simulink model "mainEthan"  (R2023b)
settings: Solver=ode113  StartTime=tstart  StopTime=tend  RelTol=relTol  AbsTol=absTol
values from neighbouring files (symbols this model uses):
  DCM_initial = targetDCM([26321453.5527815,	-132781955.130633,	-57571626.5531097]', R_princ)    [EulerEquations.m]    (also in main_script.m)
  inertia_p = [85.075, 0, 0; 0, 85.075, 0; 0, 0, 120.2515]    [omega_dot.m]
  omega_init = [0; 0; 0.01]    [EulerEquations.m]    (also in main_script.m)
  state_ECI_init = [R_PQW_IJK*state_PQW_init(1:3)';R_PQW_IJK*state_PQW_init(4:6)']    [OrbitPropagation.m]
  theta = UT1_to_theta(UT1)    [EulerEquations.m]    (also in UT1_to_theta.m = rotz(-GMST*180/pi); main_script.m)
  tstart = 0    [EulerEquations.m]    (also in main_script.m)
  UT1 = [1,25,2004,00]    [EulerEquations.m]    (also in main_script.m)
undefined symbols (not defined in the file or in its folder): A, A_star, I_w, max_dipole, max_wheel_om, max_wheel_torque, omega_w_init, R_princ
libraries: simulink x4, dspmathops x3, aerolibatmos2 x1, matrix_library x1
(part 1 of 2)
settings Model: Creator=Anna  LastModifiedBy=Anna

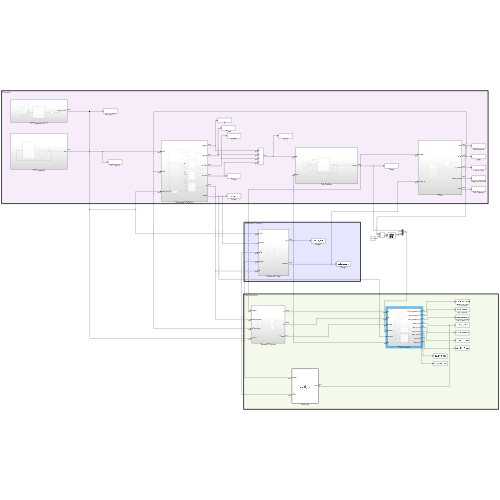
[thumbnail: Simulink's stored preview of the top-level diagram]
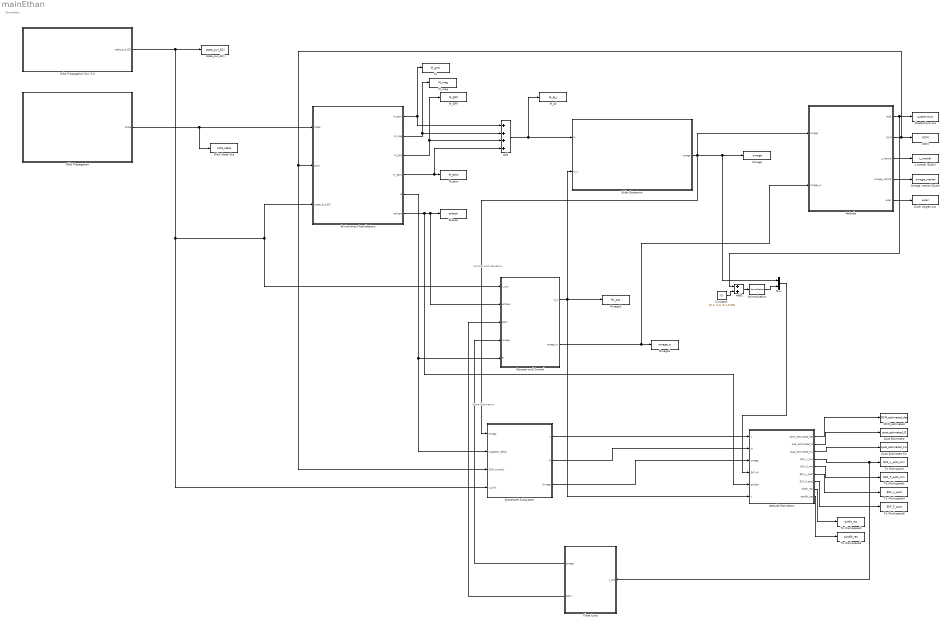
== system mainEthan ==
  note: Control and Actuation
  note: Simulation
  note: State Estimation
  Actuator and Control : Subsystem
  Add : Sum  Inputs=++++
  Add1 : Sum
  Attitude : Subsystem
  Attitude Estimation : Subsystem
  Close Loop : MATLAB Function  TreatAsAtomicUnit=on
  Constant : Constant  Value=[0.1, 0.2, 0.1,0.05]
  DCM : ToWorkspace  VariableName=DCM  SaveFormat=Timeseries  SampleTime=-1
  DCM_estimated : ToWorkspace  VariableName=DCM_estimated_det  SaveFormat=Timeseries  SampleTime=-1
      settings: Save2DSignal=2-D array (concatenate along first dimension)
  Eclipse : ToWorkspace  VariableName=eclipse  SaveFormat=Timeseries  SampleTime=-1
  Environment Petrubations : Subsystem
  Euler Angles out : ToWorkspace  VariableName=euler  SaveFormat=Timeseries  SampleTime=-1
  Euler Equations : Subsystem
  L inertial (Euler) : ToWorkspace  VariableName=L_inertial  SaveFormat=Timeseries  SampleTime=-1
  M : ToWorkspace  VariableName=M_grav  SaveFormat=Timeseries  SampleTime=-1
      settings: Save2DSignal=2-D array (concatenate along first dimension)
  M_All : ToWorkspace  VariableName=M_ALL  SaveFormat=Timeseries  SampleTime=-1
      settings: Save2DSignal=2-D array (concatenate along first dimension)
  M_SRP : ToWorkspace  VariableName=M_SRP  SaveFormat=Timeseries  SampleTime=-1
      settings: Save2DSignal=2-D array (concatenate along first dimension)
  M_aero : ToWorkspace  VariableName=M_aero  SaveFormat=Timeseries  SampleTime=-1
      settings: Save2DSignal=2-D array (concatenate along first dimension)
  M_mag : ToWorkspace  VariableName=M_mag  SaveFormat=Timeseries  SampleTime=-1
      settings: Save2DSignal=2-D array (concatenate along first dimension)
  Mux : Mux  Inputs=2
  Normalization : dspmathops/Normalization  NormType=Squared 2-norm  Bias=1e-10  NormOver=Each column  Dimension=1  roundingMode=Floor  overflowMode=off  accumDataTypeStr=Inherit: Same as product output  accumLastDataTypeStr=Inherit: Same as product output  outputDataTypeStr=Inherit: Same as product output  outputMin=[]  outputMax=[]  outputLastDataTypeStr=Inherit: Same as product output
  Omega : ToWorkspace  VariableName=omega  SaveFormat=Timeseries  SampleTime=-1
      settings: Save2DSignal=2-D array (concatenate along first dimension)
  Omega inertial (Euler) : ToWorkspace  VariableName=omega_inertial  SaveFormat=Timeseries  SampleTime=-1
  Omega1 : ToWorkspace  VariableName=omega_w  SaveFormat=Timeseries  SampleTime=-1
      settings: Save2DSignal=2-D array (concatenate along first dimension)
  Omega2 : ToWorkspace  VariableName=Mc_act  SaveFormat=Timeseries  SampleTime=-1
      settings: Save2DSignal=2-D array (concatenate along first dimension)
  Orbit Propagation : Subsystem
  Orbit Propagation Sun 3.0 : Subsystem
  Orbit State Out : ToWorkspace  VariableName=orbit_state  SaveFormat=Timeseries  SampleTime=-1
  Quat Estimated : ToWorkspace  VariableName=quat_estimated_Q  SaveFormat=Timeseries  SampleTime=-1
  Quat Estimated Kin : ToWorkspace  VariableName=quat_estimated_kin  SaveFormat=Timeseries  SampleTime=-1
  Quaternions out : ToWorkspace  VariableName=quaternions  SaveFormat=Timeseries  SampleTime=-1
  Spacecraft Subsystem : Subsystem
  To Workspace : ToWorkspace  VariableName=EKF_x_post_min  SaveFormat=Timeseries  SampleTime=-1
  To Workspace1 : ToWorkspace  VariableName=EKF_P_post_min  SaveFormat=Timeseries  SampleTime=-1
  To Workspace2 : ToWorkspace  VariableName=prefit_res  SaveFormat=Timeseries  SampleTime=-1
  To Workspace3 : ToWorkspace  VariableName=postfit_res  SaveFormat=Timeseries  SampleTime=-1
  To Workspace4 : ToWorkspace  VariableName=EKF_x_post  SaveFormat=Timeseries  SampleTime=-1
  To Workspace5 : ToWorkspace  VariableName=EKF_P_post  SaveFormat=Timeseries  SampleTime=-1
  state_sun_ECI : ToWorkspace  VariableName=state_sun_ECI  SaveFormat=Timeseries  SampleTime=-1
  wires:
  Environment Petrubations/2(M_mag) -> M_mag/1, Add/2
  Orbit Propagation/1(state) -> Orbit State Out/1, Environment Petrubations/1(state)
  Add/1 -> Euler Equations/1(M), M_All/1
  Environment Petrubations/3(M_SRP) -> M_SRP/1, Add/3
  Environment Petrubations/4(M_aero) -> Add/4, M_aero/1
  Orbit Propagation Sun 3.0/1(state_sun_ECI) -> Spacecraft Subsystem/4(r_sun1), Environment Petrubations/3(state_Sun_ECI), Actuator and Control/1(r_sun), state_sun_ECI/1
  Spacecraft Subsystem/1(V) -> Attitude Estimation/1(V)
  Spacecraft Subsystem/2(M) -> Attitude Estimation/2(M)
  Environment Petrubations/5(B) -> Spacecraft Subsystem/2(magnetic_field1), Actuator and Control/5(B)
  Attitude Estimation/1(DCM_estimated_det) -> DCM_estimated/1
  Attitude Estimation/2(quat_estimated_Q) -> Quat Estimated/1
  Attitude Estimation/3(quat_estimated_kin) -> Quat Estimated Kin/1
  Spacecraft Subsystem/3(Omega) -> Attitude Estimation/3(omega)
  Attitude Estimation/5(EKF_P_min) -> To Workspace1/1
  Attitude Estimation/4(EKF_x_min) -> To Workspace/1, Close Loop/1(x_est)
  Mux/1 -> Attitude Estimation/4(EKF x0)
  Attitude Estimation/7(EKF_P_post) -> To Workspace5/1
  Attitude Estimation/6(EKF_x_post) -> To Workspace4/1
  Environment Petrubations/6(eclipse) -> Attitude Estimation/5(" eclipse"), Actuator and Control/2(eclipse), Eclipse/1
  Attitude Estimation/8(prefit_res) -> To Workspace2/1
  Attitude Estimation/9(postfit_res) -> To Workspace3/1
  Normalization/1 -> Mux/2
  Add1/1 -> Normalization/1
  Constant/1 -> Add1/2
  Actuator and Control/1(M_c) -> Euler Equations/2(M_c), Omega2/1, Attitude Estimation/6(u)
  Actuator and Control/2(omega_w) -> Attitude/2(omega_w), Omega1/1
  Close Loop/1(omega) -> Actuator and Control/4(omega)
  Close Loop/2(DCM) -> Actuator and Control/3(DCM)
  Environment Petrubations/1(M_grav) -> Add/1, M/1
  Attitude/2(DCM) -> DCM/1, Spacecraft Subsystem/3(DCM current1), Environment Petrubations/2(DCM)
  Attitude/1(quat) -> Quaternions out/1, Add1/1
  Euler Equations/1(omega) -> Attitude/1(omega), Omega/1, Mux/1, Spacecraft Subsystem/1(omega)
  Attitude/3(L_inertial) -> L inertial (Euler)/1
  Attitude/4(omega_inertial) -> Omega inertial (Euler)/1
  Attitude/5(euler) -> Euler Angles out/1

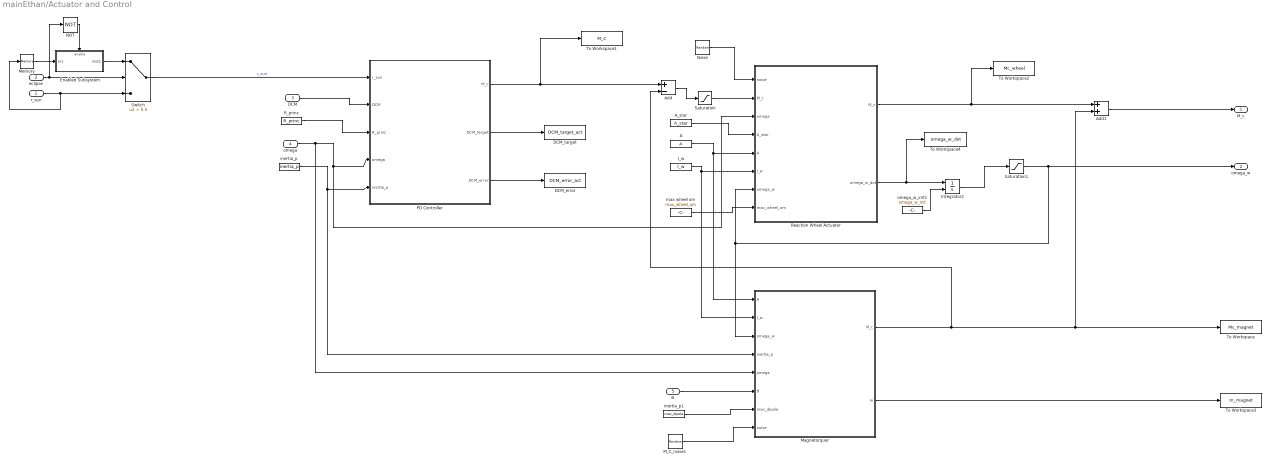
== system mainEthan/Actuator and Control ==
  r_sun : Inport
  eclipse : Inport  Port=2
  DCM : Inport  Port=3
  omega : Inport  Port=4
  B : Inport  Port=5
  A : Constant  Value=A
  A_star : Constant  Value=A_star
  Add : Sum  Inputs=+-
  Add1 : Sum
  DCM_error : ToWorkspace  VariableName=DCM_error_act  SaveFormat=Timeseries  SampleTime=-1
      settings: Save2DSignal=2-D array (concatenate along first dimension)
  DCM_target : ToWorkspace  VariableName=DCM_target_act  SaveFormat=Timeseries  SampleTime=-1
      settings: Save2DSignal=2-D array (concatenate along first dimension)
  Enabled Subsystem : Subsystem  TreatAsAtomicUnit=on
  I_w : Constant  Value=I_w
  Integrator2 : Integrator  InitialConditionSource=external  AbsoluteTolerance=absTol
  M_C_noise1 : RandomNumber  Variance=(0.00005/166)*2  Seed=[130,131,132]  SampleTime=0.1  VectorParams1D=off
  Magnetorquer : MATLAB Function  TreatAsAtomicUnit=on
  Memory : Memory  InitialCondition=[0;0;0]
  NOT : Logic  Operator=NOT  IconShape=distinctive  AllPortsSameDT=off  OutDataTypeStr=boolean
  Noise : RandomNumber  Variance=(0.00005/166)*2  Seed=[120,121,122, 123]  SampleTime=0.1  VectorParams1D=off
  PD Controller : MATLAB Function  TreatAsAtomicUnit=on
  R_princ : Constant  Value=R_princ
  Reaction Wheel Actuator : MATLAB Function  TreatAsAtomicUnit=on
  Saturation : Saturate  UpperLimit=max_wheel_torque  LowerLimit=-max_wheel_torque
  Saturation1 : Saturate  UpperLimit=max_wheel_om  LowerLimit=-max_wheel_om
  Switch : Switch  Criteria=u2 > Threshold  Threshold=0.5  SaturateOnIntegerOverflow=off  InputSameDT=off
  To Workspace : ToWorkspace  VariableName=Mc_magnet  SaveFormat=Timeseries  SampleTime=-1
  To Workspace1 : ToWorkspace  VariableName=M_C  SaveFormat=Timeseries  SampleTime=-1
  To Workspace2 : ToWorkspace  VariableName=Mc_wheel  SaveFormat=Timeseries  SampleTime=-1
  To Workspace3 : ToWorkspace  VariableName=m_magnet  SaveFormat=Timeseries  SampleTime=-1
  To Workspace4 : ToWorkspace  VariableName=omega_w_dot  SaveFormat=Timeseries  SampleTime=-1
  inertia_p : Constant  Value=inertia_p
  inertia_p1 : Constant  Value=max_dipole
  max wheel om : Constant  Value=max_wheel_om
  omega_w_init1 : Constant  Value=omega_w_init  VectorParams1D=off
  M_c : Outport
  omega_w : Outport  Port=2
  wires:
  omega_w_init1/1 -> Integrator2/2
  PD Controller/2(DCM_target) -> DCM_target/1
  omega/1 -> Reaction Wheel Actuator/3(omega), PD Controller/4(omega), Magnetorquer/5(omega)
  R_princ/1 -> PD Controller/3(R_princ)
  inertia_p/1 -> Magnetorquer/4(inertia_p), PD Controller/5(inertia_p)
  DCM/1 -> PD Controller/2(DCM)
  A_star/1 -> Reaction Wheel Actuator/4(A_star)
  PD Controller/3(DCM_error) -> DCM_error/1
  Reaction Wheel Actuator/2(omega_w_dot) -> To Workspace4/1, Integrator2/1
  Integrator2/1 -> Saturation1/1
  I_w/1 -> Reaction Wheel Actuator/6(I_w), Magnetorquer/2(I_w)
  A/1 -> Magnetorquer/1(A), Reaction Wheel Actuator/5(A)
  B/1 -> Magnetorquer/6(B)
  Magnetorquer/2(m) -> To Workspace3/1
  Switch/1 -> PD Controller/1(r_sun)  "r_sun"
  r_sun/1 -> Memory/1, Switch/3
  eclipse/1 -> NOT/1, Switch/2
  Memory/1 -> Enabled Subsystem/1(In1)
  Enabled Subsystem/1(Out1) -> Switch/1
  NOT/1 -> Enabled Subsystem/Enable
  PD Controller/1(M_c) -> Add/1, To Workspace1/1
  Saturation/1 -> Reaction Wheel Actuator/2("M_c ")
  Saturation1/1 -> omega_w/1, Magnetorquer/3(omega_w), Reaction Wheel Actuator/7(omega_w)
  max wheel om/1 -> Reaction Wheel Actuator/8(max_wheel_om)
  Add/1 -> Saturation/1
  Add1/1 -> M_c/1
  Reaction Wheel Actuator/1(M_c) -> To Workspace2/1, Add1/1
  Magnetorquer/1(M_c) -> Add/2, Add1/2, To Workspace/1
  inertia_p1/1 -> Magnetorquer/7(max_dipole)
  Noise/1 -> Reaction Wheel Actuator/1(noise)
  M_C_noise1/1 -> Magnetorquer/8(noise)

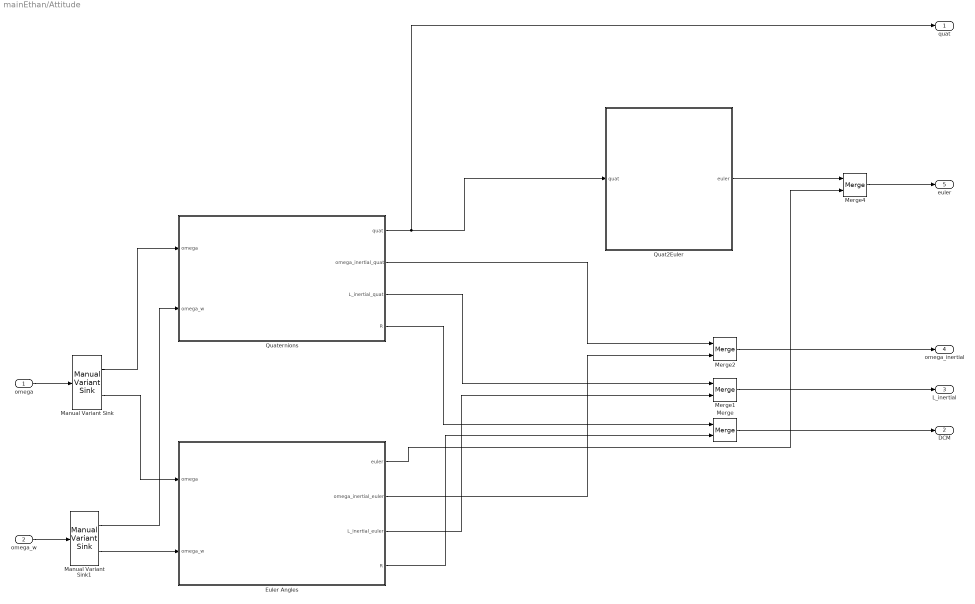
== system mainEthan/Attitude ==
  omega : Inport
  omega_w : Inport  Port=2
  Euler Angles : Subsystem
  Manual Variant Sink : simulink/Signal Routing/Manual Variant Sink  NumChoices=2  LabelModeActiveChoice=V_1
  Manual Variant Sink1 : simulink/Signal Routing/Manual Variant Sink  NumChoices=2  LabelModeActiveChoice=V_1
  Merge{,1..2,4} (4 alike) : Merge
  Quat2Euler : MATLAB Function  TreatAsAtomicUnit=on
  Quaternions : Subsystem
  quat : Outport
  DCM : Outport  Port=2
  L_inertial : Outport  Port=3
  omega_inertial : Outport  Port=4
  euler : Outport  Port=5
  wires:
  Merge/1 -> DCM/1
  omega/1 -> Manual Variant Sink/1
  omega_w/1 -> Manual Variant Sink1/1
  Quaternions/1(quat) -> quat/1, Quat2Euler/1(quat)
  Euler Angles/1(euler) -> Merge4/2
  Euler Angles/3(L_inertial_euler) -> Merge1/2
  Quat2Euler/1(euler) -> Merge4/1
  Manual Variant Sink1/1 -> Quaternions/2(omega_w)
  Manual Variant Sink1/2 -> Euler Angles/2(omega_w)
  Euler Angles/4(R) -> Merge/2
  Manual Variant Sink/1 -> Quaternions/1(omega)
  Quaternions/4(R) -> Merge/1
  Quaternions/3(L_inertial_quat) -> Merge1/1
  Manual Variant Sink/2 -> Euler Angles/1(omega)
  Merge1/1 -> L_inertial/1
  Merge2/1 -> omega_inertial/1
  Merge4/1 -> euler/1
  Quaternions/2(omega_inertial_quat) -> Merge2/1
  Euler Angles/2(omega_inertial_euler) -> Merge2/2

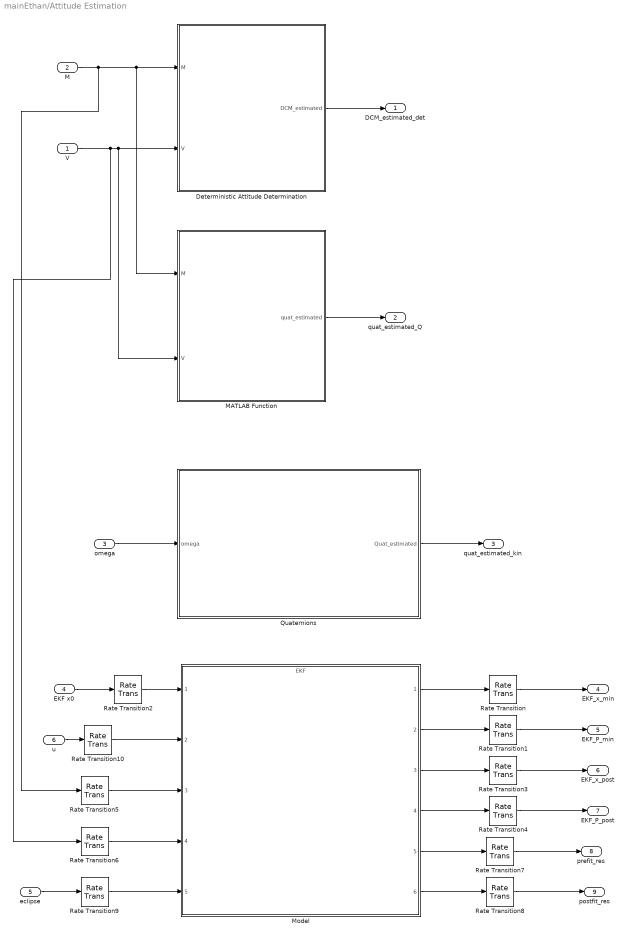
== system mainEthan/Attitude Estimation ==
  V : Inport
  M : Inport  Port=2
  omega : Inport  Port=3
  EKF x0 : Inport  Port=4
  " eclipse" : Inport  Port=5  PortDimensions=1
  u : Inport  Port=6
  Deterministic Attitude Determination : MATLAB Function  TreatAsAtomicUnit=on
  MATLAB Function : MATLAB Function  TreatAsAtomicUnit=on
  Model : ModelReference  ModelNameDialog=EKF.slx  SimulationMode=Normal  ModelReferenceVersion=1.144
  Quaternions : Subsystem
  Rate Transition{,1..10} (11 alike) : RateTransition
  DCM_estimated_det : Outport
  quat_estimated_Q : Outport  Port=2
  quat_estimated_kin : Outport  Port=3
  EKF_x_min : Outport  Port=4
  EKF_P_min : Outport  Port=5
  EKF_x_post : Outport  Port=6
  EKF_P_post : Outport  Port=7
  prefit_res : Outport  Port=8
  postfit_res : Outport  Port=9
  wires:
  Deterministic Attitude Determination/1(DCM_estimated) -> DCM_estimated_det/1
  MATLAB Function/1(quat_estimated) -> quat_estimated_Q/1
  M/1 -> Rate Transition5/1, MATLAB Function/1(M), Deterministic Attitude Determination/1(M)
  Quaternions/1(Quat_estimated) -> quat_estimated_kin/1
  V/1 -> Rate Transition6/1, MATLAB Function/2(V), Deterministic Attitude Determination/2(V)
  omega/1 -> Quaternions/1(omega)
  Model/1 -> Rate Transition/1
  Rate Transition/1 -> EKF_x_min/1
  Model/2 -> Rate Transition1/1
  Rate Transition1/1 -> EKF_P_min/1
  EKF x0/1 -> Rate Transition2/1
  Rate Transition2/1 -> Model/1
  Model/3 -> Rate Transition3/1
  Model/4 -> Rate Transition4/1
  Rate Transition4/1 -> EKF_P_post/1
  Rate Transition3/1 -> EKF_x_post/1
  Rate Transition5/1 -> Model/3
  Rate Transition6/1 -> Model/4
  Rate Transition7/1 -> prefit_res/1
  Model/5 -> Rate Transition7/1
  Rate Transition8/1 -> postfit_res/1
  Model/6 -> Rate Transition8/1
  Rate Transition9/1 -> Model/5
  " eclipse"/1 -> Rate Transition9/1
  Rate Transition10/1 -> Model/2
  u/1 -> Rate Transition10/1

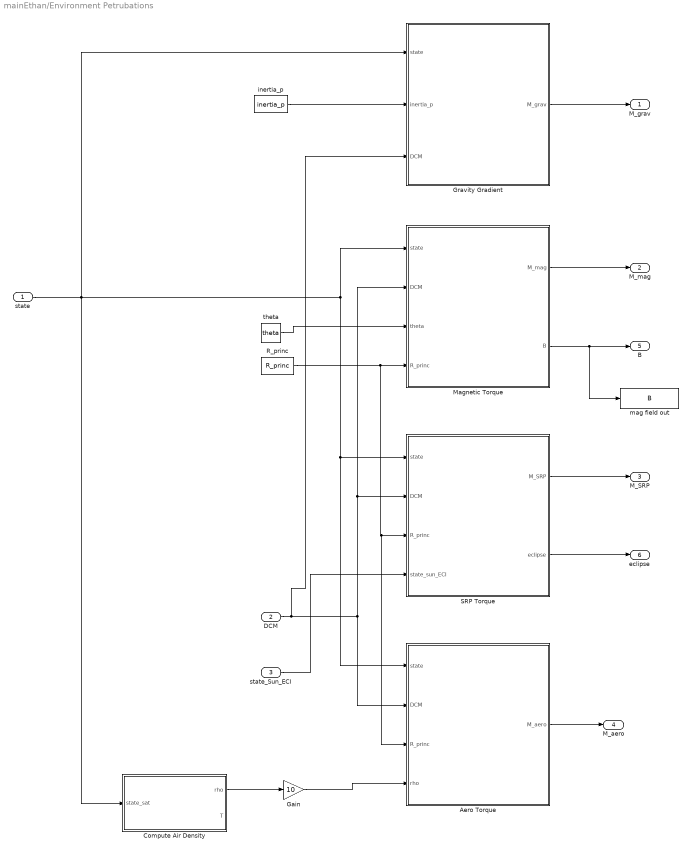
== system mainEthan/Environment Petrubations ==
  state : Inport
  DCM : Inport  Port=2
  state_Sun_ECI : Inport  Port=3
  Aero Torque : MATLAB Function  TreatAsAtomicUnit=on
  Compute Air Density : Subsystem
  Gain : Gain  Gain=10
  Gravity Gradient : MATLAB Function  TreatAsAtomicUnit=on
  Magnetic Torque : MATLAB Function  TreatAsAtomicUnit=on
  R_princ : Constant  Value=R_princ
  SRP Torque : MATLAB Function  TreatAsAtomicUnit=on
  inertia_p : Constant  Value=inertia_p
  mag field out : ToWorkspace  VariableName=B  SaveFormat=Timeseries  SampleTime=-1
  theta : Constant  Value=theta
  M_grav : Outport
  M_mag : Outport  Port=2
  M_SRP : Outport  Port=3
  M_aero : Outport  Port=4
  B : Outport  Port=5
  eclipse : Outport  Port=6
  wires:
  Magnetic Torque/1(M_mag) -> M_mag/1
  SRP Torque/1(M_SRP) -> M_SRP/1
  state/1 -> Magnetic Torque/1(state), Aero Torque/1(state), SRP Torque/1(state), Gravity Gradient/1(state), Compute Air Density/1(state_sat)
  DCM/1 -> Gravity Gradient/3(DCM), Aero Torque/2(DCM), Magnetic Torque/2(DCM), SRP Torque/2(DCM)
  theta/1 -> Magnetic Torque/3(theta)
  R_princ/1 -> Aero Torque/3(R_princ), SRP Torque/3(R_princ), Magnetic Torque/4(R_princ)
  state_Sun_ECI/1 -> SRP Torque/4(state_sun_ECI)
  Aero Torque/1(M_aero) -> M_aero/1
  SRP Torque/2(eclipse) -> eclipse/1
  Magnetic Torque/2(B) -> mag field out/1, B/1
  Gain/1 -> Aero Torque/4(rho)
  Compute Air Density/1(rho) -> Gain/1
  Gravity Gradient/1(M_grav) -> M_grav/1
  inertia_p/1 -> Gravity Gradient/2(inertia_p)

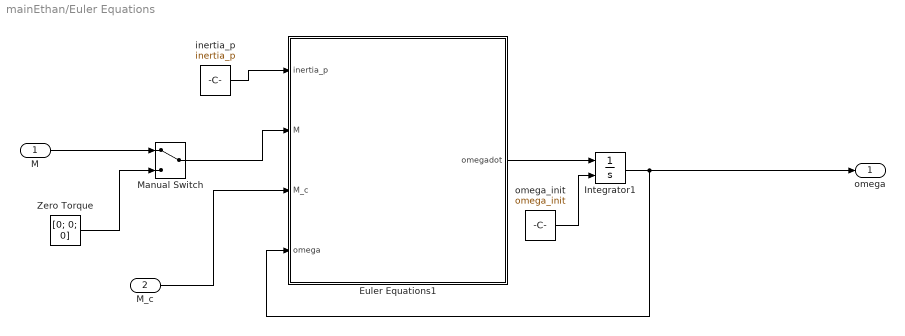
== system mainEthan/Euler Equations ==
  M : Inport
  M_c : Inport  Port=2
  Euler Equations1 : MATLAB Function  TreatAsAtomicUnit=on
  Integrator1 : Integrator  InitialConditionSource=external  AbsoluteTolerance=absTol
  Manual Switch : ManualSwitch
  Zero Torque : Constant  Value=[0; 0; 0]
  inertia_p : Constant  Value=inertia_p
  omega_init : Constant  Value=omega_init  VectorParams1D=off
  omega : Outport
  wires:
  inertia_p/1 -> Euler Equations1/1(inertia_p)
  Euler Equations1/1(omegadot) -> Integrator1/1
  Integrator1/1 -> omega/1, Euler Equations1/4(omega)
  omega_init/1 -> Integrator1/2
  Manual Switch/1 -> Euler Equations1/2(M)
  M/1 -> Manual Switch/1
  Zero Torque/1 -> Manual Switch/2
  M_c/1 -> Euler Equations1/3(M_c)

== system mainEthan/Orbit Propagation ==
  Integrator3 : Integrator  InitialConditionSource=external  AbsoluteTolerance=absTol
  Orbit Propagation1 : MATLAB Function  TreatAsAtomicUnit=on
  initial state ECI : Constant  Value=state_ECI_init
  state : Outport
  wires:
  initial state ECI/1 -> Integrator3/2
  Orbit Propagation1/1(statedot) -> Integrator3/1
  Integrator3/1 -> state/1, Orbit Propagation1/1(state)

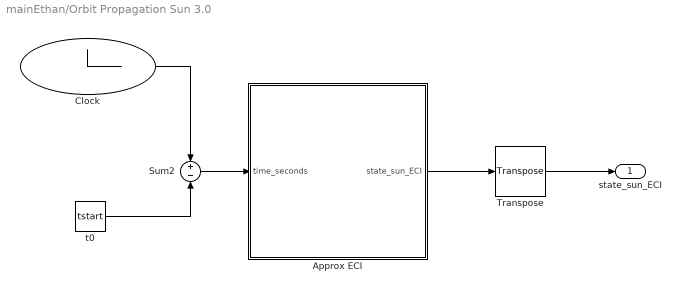
== system mainEthan/Orbit Propagation Sun 3.0 ==
  Approx ECI : MATLAB Function  TreatAsAtomicUnit=on
  Clock : Clock
  Sum2 : Sum  Inputs=+-
  Transpose : matrix_library/Transpose
  t0 : Constant  Value=tstart
  state_sun_ECI : Outport
  wires:
  Clock/1 -> Sum2/1
  t0/1 -> Sum2/2
  Sum2/1 -> Approx ECI/1(time_seconds)
  Transpose/1 -> state_sun_ECI/1
  Approx ECI/1(state_sun_ECI) -> Transpose/1

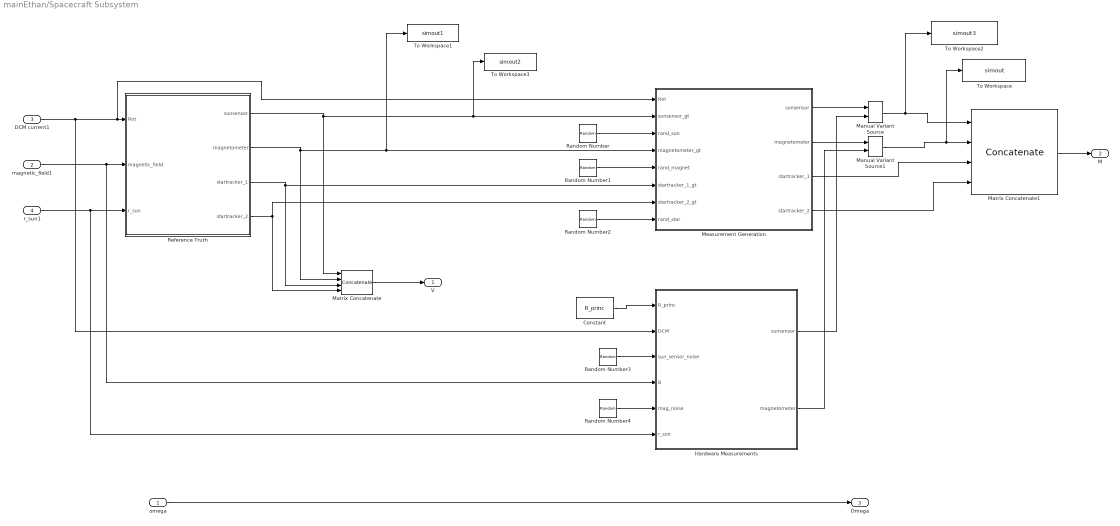
== system mainEthan/Spacecraft Subsystem ==
  omega : Inport
  magnetic_field1 : Inport  Port=2
  DCM current1 : Inport  Port=3
  r_sun1 : Inport  Port=4
  Constant : Constant  Value=R_princ
  Hardware Measurements : MATLAB Function  TreatAsAtomicUnit=on
  Manual Variant Source : simulink/Signal Routing/Manual Variant Source  NumChoices=2  LabelModeActiveChoice=V_2
  Manual Variant Source1 : simulink/Signal Routing/Manual Variant Source  NumChoices=2  LabelModeActiveChoice=V_2
  Matrix Concatenate : Concatenate  NumInputs=4  Mode=Multidimensional array  ConcatenateDimension=2
  Matrix Concatenate1 : Concatenate  NumInputs=4  Mode=Multidimensional array  ConcatenateDimension=2
  Measurement Generation : MATLAB Function  TreatAsAtomicUnit=on
  Random Number : RandomNumber  Variance=0.5  Seed=[80, 81]  SampleTime=0.1
  Random Number1 : RandomNumber  Variance=0.0075*65*10^-6  Seed=[70, 71, 72]  SampleTime=0.1
  Random Number2 : RandomNumber  Variance=5/3600  Seed=[0, 1,2,3,4,5,6,7,8,9,10,11,12,13,14; 15,16,17,18,19,20,21,22,23,24,25,26,27,28,29; 30, 31, 32,33,34,35,36,37,38,39,40,41,42,43,44;45,46,47,48,49,50,51,52,53,54,55,56,57,58,59]  SampleTime=0.1
  Random Number3 : RandomNumber  Variance=.0025  Seed=91  SampleTime=0.1
  Random Number4 : RandomNumber  Variance=100*((10^-6)/(10^-9))*12*10^-12  Seed=[95, 96, 97]  SampleTime=0.1
  Reference Truth : MATLAB Function  TreatAsAtomicUnit=on
  To Workspace : ToWorkspace  VariableName=simout  SaveFormat=Timeseries  SampleTime=-1
  To Workspace1 : ToWorkspace  VariableName=simout1  SaveFormat=Timeseries  SampleTime=-1
  To Workspace2 : ToWorkspace  VariableName=simout3  SaveFormat=Timeseries  SampleTime=-1
  To Workspace3 : ToWorkspace  VariableName=simout2  SaveFormat=Timeseries  SampleTime=-1
  V : Outport
  M : Outport  Port=2
  Omega : Outport  Port=3
  wires:
  r_sun1/1 -> Reference Truth/3(r_sun), Hardware Measurements/6(r_sun)
  magnetic_field1/1 -> Hardware Measurements/4(B), Reference Truth/2(magnetic_field)
  DCM current1/1 -> Hardware Measurements/2(DCM), Measurement Generation/1(Rot), Reference Truth/1(Rot)
  Matrix Concatenate1/1 -> M/1
  Matrix Concatenate/1 -> V/1
  Reference Truth/1(sunsensor) -> Matrix Concatenate/1, To Workspace3/1, Measurement Generation/2(sunsensor_gt)
  Reference Truth/3(startracker_1) -> Measurement Generation/6(startracker_1_gt), Matrix Concatenate/3
  Reference Truth/4(startracker_2) -> Measurement Generation/7(startracker_2_gt), Matrix Concatenate/4
  omega/1 -> Omega/1
  Random Number/1 -> Measurement Generation/3(rand_sun)
  Random Number1/1 -> Measurement Generation/5(rand_magnet)
  Random Number2/1 -> Measurement Generation/8(rand_star)
  Measurement Generation/4(startracker_2) -> Matrix Concatenate1/4
  Reference Truth/2(magnetometer) -> To Workspace1/1, Measurement Generation/4(magnetometer_gt), Matrix Concatenate/2
  Measurement Generation/3(startracker_1) -> Matrix Concatenate1/3
  Constant/1 -> Hardware Measurements/1(R_princ)
  Random Number3/1 -> Hardware Measurements/3(sun_sensor_noise)
  Manual Variant Source/1 -> To Workspace2/1, Matrix Concatenate1/1
  Measurement Generation/1(sunsensor) -> Manual Variant Source/1
  Hardware Measurements/1(sunsensor) -> Manual Variant Source/2
  Measurement Generation/2(magnetometer) -> Manual Variant Source1/1
  Manual Variant Source1/1 -> To Workspace/1, Matrix Concatenate1/2
  Hardware Measurements/2(magnetometer) -> Manual Variant Source1/2
  Random Number4/1 -> Hardware Measurements/5(mag_noise)

== system mainEthan/Actuator and Control/Enabled Subsystem ==
  In1 : Inport
  Enable : EnablePort
  Out1 : Outport
  wires:
  In1/1 -> Out1/1

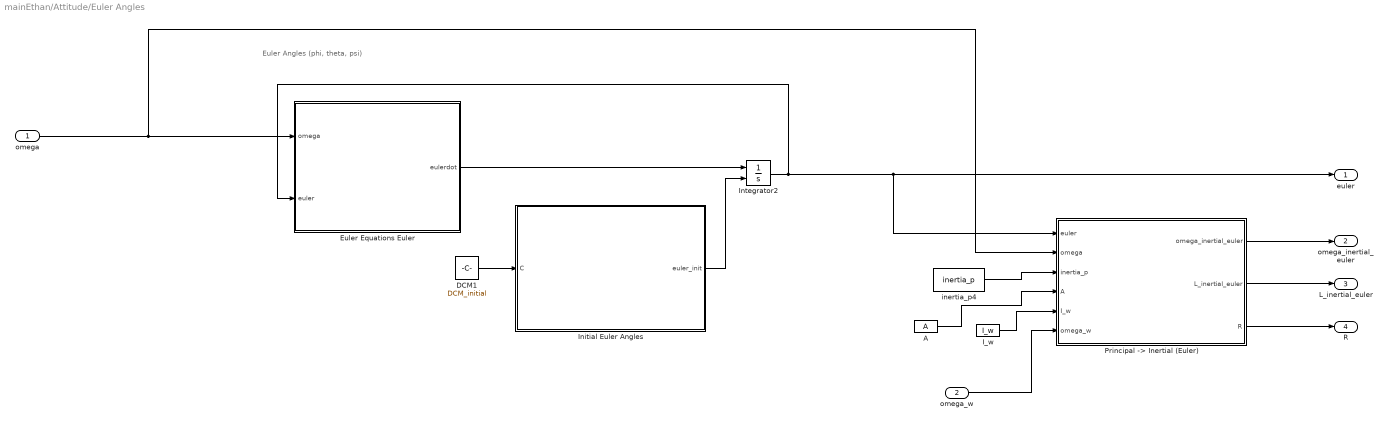
== system mainEthan/Attitude/Euler Angles ==
  note: Euler Angles (phi, theta, psi)
  omega : Inport
  omega_w : Inport  Port=2
  A : Constant  Value=A
  DCM1 : Constant  Value=DCM_initial
  Euler Equations Euler : MATLAB Function  TreatAsAtomicUnit=on
  I_w : Constant  Value=I_w
  Initial Euler Angles : MATLAB Function  TreatAsAtomicUnit=on
  Integrator2 : Integrator  InitialConditionSource=external  AbsoluteTolerance=absTol
  "Principal -> Inertial (Euler)" : MATLAB Function  TreatAsAtomicUnit=on
  inertia_p4 : Constant  Value=inertia_p
  euler : Outport
  omega_inertial_euler : Outport  Port=2
  L_inertial_euler : Outport  Port=3
  R : Outport  Port=4
  wires:
  "Principal -> Inertial (Euler)"/2(L_inertial_euler) -> L_inertial_euler/1
  Initial Euler Angles/1(euler_init) -> Integrator2/2
  "Principal -> Inertial (Euler)"/1(omega_inertial_euler) -> omega_inertial_euler/1
  "Principal -> Inertial (Euler)"/3(R) -> R/1
  Integrator2/1 -> euler/1, "Principal -> Inertial (Euler)"/1(euler), Euler Equations Euler/2(euler)
  Euler Equations Euler/1(eulerdot) -> Integrator2/1
  omega/1 -> "Principal -> Inertial (Euler)"/2(omega), Euler Equations Euler/1(omega)
  inertia_p4/1 -> "Principal -> Inertial (Euler)"/3(inertia_p)
  DCM1/1 -> Initial Euler Angles/1(C)
  omega_w/1 -> "Principal -> Inertial (Euler)"/6(omega_w)
  A/1 -> "Principal -> Inertial (Euler)"/4(A)
  I_w/1 -> "Principal -> Inertial (Euler)"/5(I_w)

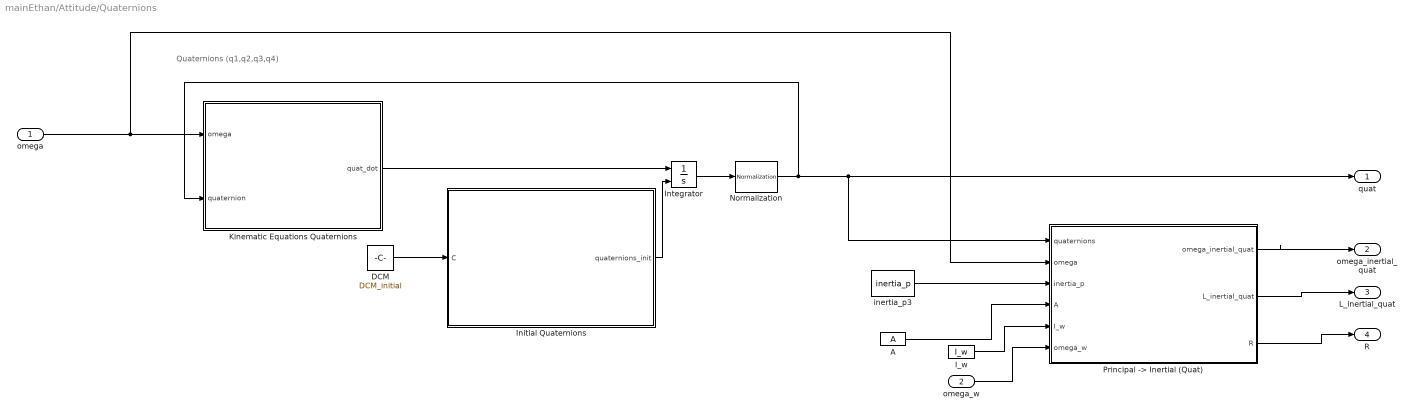
== system mainEthan/Attitude/Quaternions ==
  note: Quaternions (q1,q2,q3,q4)
  omega : Inport
  omega_w : Inport  Port=2
  A : Constant  Value=A
  DCM : Constant  Value=DCM_initial
  I_w : Constant  Value=I_w
  Initial Quaternions : MATLAB Function  TreatAsAtomicUnit=on
  Integrator : Integrator  InitialConditionSource=external  AbsoluteTolerance=absTol
  "Kinematic Equations Quaternions " : MATLAB Function  TreatAsAtomicUnit=on
  Normalization : dspmathops/Normalization  NormType=Squared 2-norm  Bias=1e-10  NormOver=Each column  Dimension=1  roundingMode=Floor  overflowMode=off  accumDataTypeStr=Inherit: Same as product output  accumLastDataTypeStr=Inherit: Same as product output  outputDataTypeStr=Inherit: Same as product output  outputMin=[]  outputMax=[]  outputLastDataTypeStr=Inherit: Same as product output
  "Principal -> Inertial (Quat)" : MATLAB Function  TreatAsAtomicUnit=on
  inertia_p3 : Constant  Value=inertia_p
  quat : Outport
  omega_inertial_quat : Outport  Port=2
  L_inertial_quat : Outport  Port=3
  R : Outport  Port=4
  wires:
  omega/1 -> "Kinematic Equations Quaternions "/1(omega), "Principal -> Inertial (Quat)"/2(omega)
  DCM/1 -> Initial Quaternions/1(C)
  "Principal -> Inertial (Quat)"/2(L_inertial_quat) -> L_inertial_quat/1
  "Kinematic Equations Quaternions "/1(quat_dot) -> Integrator/1
  "Principal -> Inertial (Quat)"/3(R) -> R/1
  Initial Quaternions/1(quaternions_init) -> Integrator/2
  Integrator/1 -> Normalization/1
  inertia_p3/1 -> "Principal -> Inertial (Quat)"/3(inertia_p)
  "Principal -> Inertial (Quat)"/1(omega_inertial_quat) -> omega_inertial_quat/1
  Normalization/1 -> quat/1, "Principal -> Inertial (Quat)"/1(quaternions), "Kinematic Equations Quaternions "/2(quaternion)
  A/1 -> "Principal -> Inertial (Quat)"/4(A)
  omega_w/1 -> "Principal -> Inertial (Quat)"/6(omega_w)
  I_w/1 -> "Principal -> Inertial (Quat)"/5(I_w)

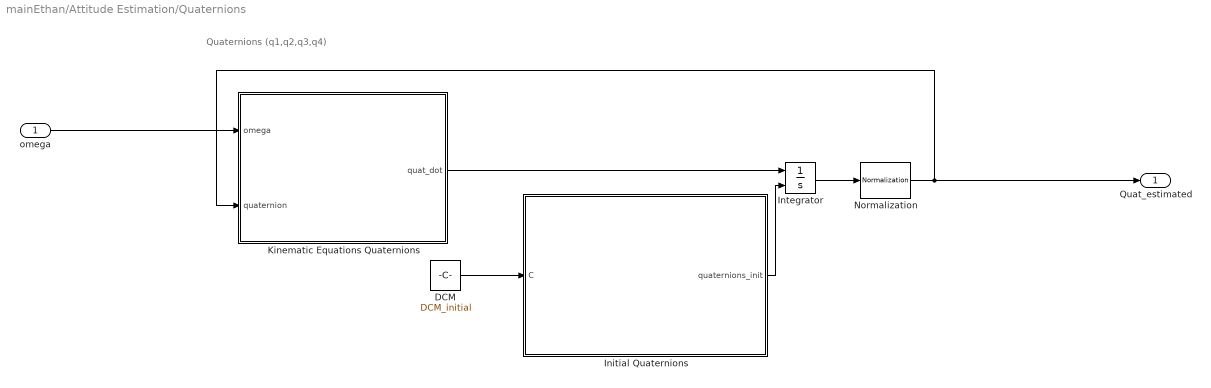
== system mainEthan/Attitude Estimation/Quaternions ==
  note: Quaternions (q1,q2,q3,q4)
  omega : Inport
  DCM : Constant  Value=DCM_initial
  Initial Quaternions : MATLAB Function  TreatAsAtomicUnit=on
  Integrator : Integrator  InitialConditionSource=external  AbsoluteTolerance=absTol
  "Kinematic Equations Quaternions " : MATLAB Function  TreatAsAtomicUnit=on
  Normalization : dspmathops/Normalization  NormType=Squared 2-norm  Bias=1e-10  NormOver=Each column  Dimension=1  roundingMode=Floor  overflowMode=off  accumDataTypeStr=Inherit: Same as product output  accumLastDataTypeStr=Inherit: Same as product output  outputDataTypeStr=Inherit: Same as product output  outputMin=[]  outputMax=[]  outputLastDataTypeStr=Inherit: Same as product output
  Quat_estimated : Outport
  wires:
  omega/1 -> "Kinematic Equations Quaternions "/1(omega)
  DCM/1 -> Initial Quaternions/1(C)
  "Kinematic Equations Quaternions "/1(quat_dot) -> Integrator/1
  Initial Quaternions/1(quaternions_init) -> Integrator/2
  Integrator/1 -> Normalization/1
  Normalization/1 -> Quat_estimated/1, "Kinematic Equations Quaternions "/2(quaternion)

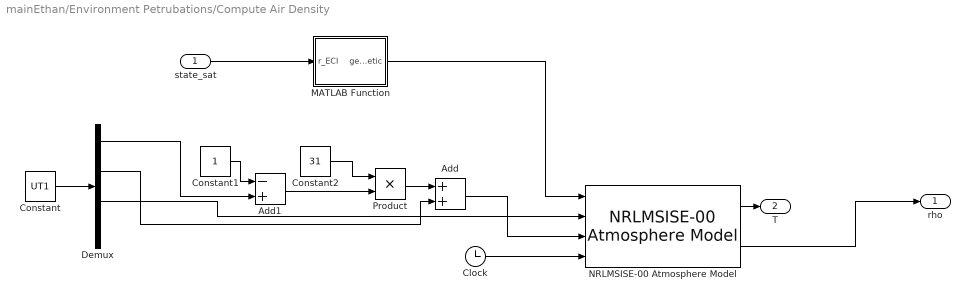
== system mainEthan/Environment Petrubations/Compute Air Density ==
  state_sat : Inport
  Add : Sum
  Add1 : Sum  Inputs=-+
  Clock : Clock
  Constant : Constant  Value=UT1
  Constant1 : Constant
  Constant2 : Constant  Value=31
  Demux : Demux
  MATLAB Function : MATLAB Function  TreatAsAtomicUnit=on
  NRLMSISE-00 Atmosphere Model : aerolibatmos2/NRLMSISE-00 Atmosphere Model  units=Metric (MKS)  lst_input=off  flux_ap_input=off  flags_input=Internal  flags=ones(1,23)  oxygen_in=off  action=Warning
  Product : Product
  rho : Outport
  T : Outport  Port=2
  wires:
  NRLMSISE-00 Atmosphere Model/1 -> T/1
  Demux/2 -> Add/2
  NRLMSISE-00 Atmosphere Model/2 -> rho/1
  Product/1 -> Add/1
  Add/1 -> NRLMSISE-00 Atmosphere Model/3
  MATLAB Function/1(geodetic) -> NRLMSISE-00 Atmosphere Model/1
  Demux/1 -> Add1/2
  Demux/3 -> NRLMSISE-00 Atmosphere Model/2
  Clock/1 -> NRLMSISE-00 Atmosphere Model/4
  Add1/1 -> Product/2
  Constant/1 -> Demux/1
  Constant2/1 -> Product/1
  state_sat/1 -> MATLAB Function/1(r_ECI)
  Constant1/1 -> Add1/1

== matlab function mainEthan/Orbit Propagation/Orbit Propagation1 ==
  data: statedot output; state input
%% return equations of motion
function statedot  = state_dot(state)
    mu = 398600.435436; %Earth centered orbit
    statedot = zeros(6, 1);
    statedot(1:3) = state(4:6);
    statedot(4:6) = -mu * state(1:3)/(norm(state(1:3))^3);
end

== matlab function mainEthan/Environment Petrubations/Gravity Gradient ==
  data: state input; inertia_p input; DCM input; M_grav output
%% return omega_dot (zero torque)
function M_grav  = gravity_gradient(state, inertia_p, DCM)
    mu = 398600.435436; %Earth centered orbit

    R_p = DCM * state(1:3);
    cx = R_p(1)/norm(R_p);
    cy = R_p(2)/norm(R_p);
    cz = R_p(3)/norm(R_p);

    M_grav = 3*mu/(norm(R_p)^3) *[(inertia_p(3,3) - inertia_p(2,2)) * cy * cz;
                    (inertia_p(1,1) - inertia_p(3,3)) * cz * cx;
                    (inertia_p(2,2) - inertia_p(1,1)) * cx * cy];
 
 
    %disp(norm(M))
end

== matlab function mainEthan/Attitude/Quat2Euler ==
  data: quat input; euler output

%% return euler angles from quaternions
function euler= quat2eul(quat)
    q0 = quat(4);
    q1 = quat(1);
    q2 = quat(2);
    q3 = quat(3);

    %123 singular for theta = 90 deg
    %phi = atan2(2*q2*q3 + 2*q0*q1, q3^2 - q2^2 - q1^2 + q0^2);
    %theta = -asin(2*q1*q3 - 2*q0*q2);
    %psi = atan2(2*q1*q2 + 2*q0*q3, q1^2 + q0^2 - q3^2 - q2^2);

    % %213 use when you rotate around y, singular for theta = 90
    phi = atan2(-2*q1*q3 + 2*q0*q2, q3^2 - q2^2 - q1^2 + q0^2);
    theta = asin(2*q2*q3 + 2*q0*q1);
    psi = atan2(-2*q1*q2 + 2*q0*q3, q2^2 - q3^2 + q0^2 - q1^2);

    %313 singular for theta = 0
    %phi = atan2(2*q1*q3 - 2*q0*q2, 2*q2*q3 + 2*q0*q1);
    %theta = acos(q3^2 - q2^2 - q1^2 + q0^2);
    %psi =atan2(2*q1*q3 + 2*q0*q2, -2*q2*q3 + 2*q0*q1);
    
    euler = [phi; theta; psi];

end

== matlab function mainEthan/Actuator and Control/PD Controller ==
  data: r_sun input; DCM input; R_princ input; M_c output; omega input; inertia_p input; DCM_target output; DCM_error output
%% return omega_dot (zero torque)
function [M_c, DCM_target, DCM_error]  = controller(r_sun, DCM, R_princ, omega, inertia_p)

    r_sun_norm = r_sun/norm(r_sun);

    %define that body x-axis will be in plane with body z-axis and r_sun
    %(perpendicular on r_sun)
    r_sun_projected = [r_sun_norm(1:2); 0];
    target_y_body = cross(r_sun_projected, r_sun_norm)./norm(cross(r_sun_projected, r_sun_norm));
    target_x_body = cross(target_y_body, r_sun_norm); %in plane

    %disp(dot(r_sun_norm, target_x_body)) %check that they are perependicular
    
    %construct target DCM in principal frame
    target_DCM = eye(3); %target DCM in principal frame
    target_DCM(1:3, 1) =  R_princ * target_x_body; %target attitude x-component principal frame
    target_DCM(1:3, 2) =  R_princ * target_y_body; %target attitude y-component principal frame
    target_DCM(1:3, 3) =  R_princ * r_sun_norm; %target attitude z-component principal frame

    DCM_target = target_DCM;
    DCM_error = DCM*DCM_target';
    n = 0.0011;
    kpx = 100*inertia_p(1,1)*n^2;
    kpy = 100*inertia_p(2,2)*n^2;
    kpz = 100*inertia_p(3,3)*n^2;

   

    kdx = 2 * 0.7 * inertia_p(1,1) * 100*n;
    kdy = 2 * 0.7 * inertia_p(2,2) * 100*n;
    kdz = 2 * 0.7 * inertia_p(3,3) * 100*n;

    
    % %Small Angle Approx
    % M_c = [0;0;0];
    % M_c(1) = - 0.5*kpx*(DCM_error(2,3) - DCM_error(3,2)) - kdx*omega(1);
    % M_c(2) = - 0.5*kpy*(DCM_error(1,3) - DCM_error(3,1)) - kdy*omega(2);
    % M_c(3) = - 0.5*kpz*(DCM_error(1,2) - DCM_error(2,1)) - kdz*omega(3);
    % 
    %213 seq
    alphay = atan2(-DCM_error(1, 3), DCM_error(3, 3));
    alphax = asin(DCM_error(2, 3));
    alphaz = atan2(-DCM_error(2, 1), DCM_error(2, 2));
    M_c = [0;0;0];
    M_c(1) = - kpx*alphax - kdx*omega(1);
    M_c(2) = - kpy*alphay- kdy*omega(2);
    M_c(3) = - kpz*alphaz - kdz*omega(3);

end

== matlab function mainEthan/Actuator and Control/Reaction Wheel Actuator ==
  data: noise input; M_c input; omega input; A_star input; A input; I_w input; omega_w input; M_c output; omega_w_dot output; max_wheel_om input
function [M_c, omega_w_dot] = RW_actuator(noise, M_c, omega, A_star, A, I_w, omega_w, max_wheel_om)
    L_w = I_w.*omega_w;
    L_w_dot = A_star * (- M_c - cross(omega,A*L_w)) + noise';
    omega_w_dot = L_w_dot./I_w;

    indices_pos_sat = (omega_w >= max_wheel_om) & (omega_w_dot > 0);
    indices_neg_sat = (omega_w <= -max_wheel_om) & (omega_w_dot < 0);
  
    omega_w_dot(indices_pos_sat | indices_neg_sat) = 0;
   

    M_c = - I_w  .* pinv(A_star) * omega_w_dot - cross(omega, A*L_w);
end

== matlab function mainEthan/Environment Petrubations/SRP Torque ==
  data: state input; DCM input; R_princ input; M_SRP output; state_sun_ECI input; eclipse output
function [M_SRP, eclipse] = SRP_torque(state, DCM, R_princ, state_sun_ECI)
    P = 1358/(3e8); % Solar Constant

    R = state(1:3)*1000; % State ECI
    R_unit = R./norm(R); % Unit State ECI
    R_E = 6378*1000; % Earth Radius

    R_Sun = state_sun_ECI; % Sun State ECI 
    R_Sun_unit = R_Sun./norm(R_Sun); % Unit Sun State ECI
    R_p_Sun = DCM * R_Sun; % Sun State Princ
    R_p_Sun_unit = R_p_Sun./norm(R_p_Sun); % Unit Sun State Princ

    M_SRP = [0;0;0];

    surface = struct('bary',[0,0,0],'size',0,'unit',[0,0,0]);

    % Eclipses
    psi = acos(dot(R_unit, R_Sun_unit));
    a_check = norm(R)*sin(psi);

    for surfacenum = 1:20
        if surfacenum == 1
            surface.bary = [-0.0129, -0.0019, 1.0022]; % Converted from cm to m
            surface.size = 0.866025; % Converted from cm² to m²
            surface.unit = [0, 0, 1];
        end
        if surfacenum == 2
            surface.bary = [-0.0129, -0.0019, -0.6008]; % Converted from cm to m
            surface.size = 0.866025; % Converted from cm² to m²
            surface.unit = [0, 0, -1];
        end
        if surfacenum == 3
            surface.bary = [0.4871, -0.0019, 0.2007]; % Converted from cm to m
            surface.size = 0.913944; % Converted from cm² to m²
            surface.unit = [1, 0, 0];
        end
        if surfacenum == 4
            surface.bary = [1.0854, -0.0019, -0.5808]; % Converted from cm to m
            surface.size = 0.690859; % Converted from cm² to m²
            surface.unit = [0, 0, 1];
        end
        if surfacenum == 5
            surface.bary = [1.0854, -0.0019, -0.6008]; % Converted from cm to m
            surface.size = 0.690859; % Converted from cm² to m²
            surface.unit = [0, 0, -1];
        end
        if surfacenum == 6
            surface.bary = [0.2371, 0.4311, 0.2007]; % Converted from cm to m
            surface.size = 0.913944; % Converted from cm² to m²
            surface.unit = [0.5, 0.866, 0];
        end
        if surfacenum == 7
            surface.bary = [0.5362, 0.9492, -0.5808]; % Converted from cm to m
            surface.size = 0.690859; % Converted from cm² to m²
            surface.unit = [0, 0, 1];
        end
        if surfacenum == 8
            surface.bary = [0.5362, 0.9492, -0.6008]; % Converted from cm to m
            surface.size = 0.690859; % Converted from cm² to m²
            surface.unit = [0, 0, -1];
        end
        if surfacenum == 9
            surface.bary = [-0.2629, 0.4311, 0.2007]; % Converted from cm to m
            surface.size = 0.913944; % Converted from cm² to m²
            surface.unit = [-0.5, 0.866, 0];
        end
        if surfacenum == 10
            surface.bary = [-0.5620, 0.9492, -0.5808]; % Converted from cm to m
            surface.size = 0.690859; % Converted from cm² to m²
            surface.unit = [0, 0, 1];
        end
        if surfacenum == 11
            surface.bary = [-0.5620, 0.9492, -0.6008]; % Converted from cm to m
            surface.size = 0.690859; % Converted from cm² to m²
            surface.unit = [0, 0, -1];
        end
        if surfacenum == 12
            surface.bary = [-0.5129, -0.0019, 0.2007]; % Converted from cm to m
            surface.size = 0.913944; % Converted from cm² to m²
            surface.unit = [-1, 0, 0];
        end
        if surfacenum == 13
            surface.bary = [-1.1111, -0.0019, -0.5808]; % Converted from cm to m
            surface.size = 0.690859; % Converted from cm² to m²
            surface.unit = [0, 0, 1];
        end
        if surfacenum == 14
            surface.bary = [-1.1111, -0.0019, -0.6008]; % Converted from cm to m
            surface.size = 0.690859; % Converted from cm² to m²
            surface.unit = [0, 0, -1];
        end
        if surfacenum == 15
            surface.bary = [-0.2629, -0.4349, 0.2007]; % Converted from cm to m
            surface.size = 0.913944; % Converted from cm² to m²
            surface.unit = [-0.5, -0.866, 0];
        end
        if surfacenum == 16
            surface.bary = [-0.5620, -0.9530, -0.5808]; % Converted from cm to m
            surface.size = 0.690859; % Converted from cm² to m²
            surface.unit = [0, 0, 1];
        end
        if surfacenum == 17
            surface.bary = [-0.5620, -0.9530, -0.6008]; % Converted from cm to m
            surface.size = 0.690859; % Converted from cm² to m²
            surface.unit = [0, 0, -1];
        end
        if surfacenum == 18
            surface.bary = [0.2371, -0.4349, 0.2007]; % Converted from cm to m
            surface.size = 0.913944; % Converted from cm² to m²
            surface.unit = [0.5, -0.866, 0];
        end
        if surfacenum == 19
            surface.bary = [0.5362, -0.9530, -0.5808]; % Converted from cm to m
            surface.size = 0.690859; % Converted from cm² to m²
            surface.unit = [0, 0, 1];
        end
        if surfacenum == 20
            surface.bary = [0.5362, -0.9530, -0.6008]; % Converted from cm to m
            surface.size = 0.690859; % Converted from cm² to m²
            surface.unit = [0, 0, -1];
        end

        bary = R_princ*(surface.bary'); % Barycenter body to princ
        A = (surface.size); % Area in m^2
        N = R_princ*(surface.unit'); % Normal vector in princ
        
        %cos_theta_StoN = dot(N,R_p_Sun_unit); % Angle between N and S vectors
        theta_StoN = acos(dot(N, R_p_Sun_unit));
        
        C_s = 0.7; % Aluminum about 70% specular reflectance 
        C_d = 0.15; 
        % 
        % disp(theta_StoN)
        % % Check if the angle is within the range of 0 to 90 degrees
        if theta_StoN >= 0 && theta_StoN <= pi/2
            e = 1; % Surfaces can see each other
        else
            e = 0; % Surfaces are obstructed
        end
        % 
        F = -P*A*cos(theta_StoN) * ((1-C_s)*R_p_Sun_unit + 2*(C_s*cos(theta_StoN) + (1/3)*C_d)*N); % Force

        M_SRP = M_SRP + e*cross(bary,F); % Summation 
    end
    eclipse = 0;
    if a_check < R_E && psi > pi/2
        eclipse = 1;
        M_SRP = [0;0;0];
    end
end

== matlab function mainEthan/Environment Petrubations/Magnetic Torque ==
  data: state input; DCM input; theta input; M_mag output; R_princ input; B output
%% return omega_dot (zero torque)
function [M_mag, B] = mag_torque(state, DCM, theta, R_princ)
    eps = 4*pi*10^-7; % Vacuum Perm
    S = 0.866025; % Surface Area inside coils, m^2
    n = 100; % Coils
    I = 35.4/25; % Current, Power/Voltage for SIM

    R = state(1:3)*1000; % State
    R_unit = R/norm(R); % Unit State
    R_E = 6378*1000; % Earth Radius
    R_p = DCM * R; % Attitude

    % Earth Mag Dipole Point Lat Long Initial
    lambda = -115.62;
    phi = 82.752;

    m_initial = R_E*[cosd(phi)*cosd(lambda);cosd(phi)*sind(lambda);sind(phi)]; % In ECEF
    m_initial = m_initial./norm(m_initial);

    m = theta*m_initial; % ECEF to ECI
    m = DCM*m; % ECI to Current Principal
    B_0 = 3.08e-5; % Earth Dipole Strength, Teslas
    
    m_sat = R_princ*[0,0,1]'; % Body to Current Principal
    m_sat = eps*S*n*I*m_sat'; % Satellite Mag Moment
    B = -((R_E^3)*B_0/(norm(R)^3)) * (3*(dot(m,R_unit))*R_unit - m); % Earth Mag Field Inertial

    M_mag = cross(m_sat,B)'; % Mag Moment
end

== matlab function mainEthan/Environment Petrubations/Aero Torque ==
  data: state input; DCM input; R_princ input; M_aero output; rho input
function M_aero = aero_torque(state, DCM, R_princ, rho)
    V = state(4:6)*1000; % Satellite Velocity
    V_p = DCM * V; % In Principal
    V_p_unit = V_p./norm(V_p); % Velocity Norm in princ

    C_d = 1.28; % Flat Plates
    % h = norm(R) - R_E; % Satellite height in meters
    % rho = 1.454*10^(-13); %(1.45e-4) * exp(-(h - 6e2) ./ 7.1835e1)
    M_aero = [0;0;0];

    rho = rho(6);

    surface = struct('bary',[0,0,0],'size',0,'unit',[0,0,0]);

    for surfacenum = 1:20
        if surfacenum == 1
            surface.bary = [-0.0129, -0.0019, 1.0022]; % Converted from cm to m
            surface.size = 0.866025; % Converted from cm² to m²
            surface.unit = [0, 0, 1];
        end
        if surfacenum == 2
            surface.bary = [-0.0129, -0.0019, -0.6008]; % Converted from cm to m
            surface.size = 0.866025; % Converted from cm² to m²
            surface.unit = [0, 0, -1];
        end
        if surfacenum == 3
            surface.bary = [0.4871, -0.0019, 0.2007]; % Converted from cm to m
            surface.size = 0.913944; % Converted from cm² to m²
            surface.unit = [1, 0, 0];
        end
        if surfacenum == 4
            surface.bary = [1.0854, -0.0019, -0.5808]; % Converted from cm to m
            surface.size = 0.690859; % Converted from cm² to m²
            surface.unit = [0, 0, 1];
        end
        if surfacenum == 5
            surface.bary = [1.0854, -0.0019, -0.6008]; % Converted from cm to m
            surface.size = 0.690859; % Converted from cm² to m²
            surface.unit = [0, 0, -1];
        end
        if surfacenum == 6
            surface.bary = [0.2371, 0.4311, 0.2007]; % Converted from cm to m
            surface.size = 0.913944; % Converted from cm² to m²
            surface.unit = [0.5, 0.866, 0];
        end
        if surfacenum == 7
            surface.bary = [0.5362, 0.9492, -0.5808]; % Converted from cm to m
            surface.size = 0.690859; % Converted from cm² to m²
            surface.unit = [0, 0, 1];
        end
        if surfacenum == 8
            surface.bary = [0.5362, 0.9492, -0.6008]; % Converted from cm to m
            surface.size = 0.690859; % Converted from cm² to m²
            surface.unit = [0, 0, -1];
        end
        if surfacenum == 9
            surface.bary = [-0.2629, 0.4311, 0.2007]; % Converted from cm to m
            surface.size = 0.913944; % Converted from cm² to m²
            surface.unit = [-0.5, 0.866, 0];
        end
        if surfacenum == 10
            surface.bary = [-0.5620, 0.9492, -0.5808]; % Converted from cm to m
            surface.size = 0.690859; % Converted from cm² to m²
            surface.unit = [0, 0, 1];
        end
        if surfacenum == 11
            surface.bary = [-0.5620, 0.9492, -0.6008]; % Converted from cm to m
            surface.size = 0.690859; % Converted from cm² to m²
            surface.unit = [0, 0, -1];
        end
        if surfacenum == 12
            surface.bary = [-0.5129, -0.0019, 0.2007]; % Converted from cm to m
            surface.size = 0.913944; % Converted from cm² to m²
            surface.unit = [-1, 0, 0];
        end
        if surfacenum == 13
            surface.bary = [-1.1111, -0.0019, -0.5808]; % Converted from cm to m
            surface.size = 0.690859; % Converted from cm² to m²
            surface.unit = [0, 0, 1];
        end
        if surfacenum == 14
            surface.bary = [-1.1111, -0.0019, -0.6008]; % Converted from cm to m
            surface.size = 0.690859; % Converted from cm² to m²
            surface.unit = [0, 0, -1];
        end
        if surfacenum == 15
            surface.bary = [-0.2629, -0.4349, 0.2007]; % Converted from cm to m
            surface.size = 0.913944; % Converted from cm² to m²
            surface.unit = [-0.5, -0.866, 0];
        end
        if surfacenum == 16
            surface.bary = [-0.5620, -0.9530, -0.5808]; % Converted from cm to m
            surface.size = 0.690859; % Converted from cm² to m²
            surface.unit = [0, 0, 1];
        end
        if surfacenum == 17
            surface.bary = [-0.5620, -0.9530, -0.6008]; % Converted from cm to m
            surface.size = 0.690859; % Converted from cm² to m²
            surface.unit = [0, 0, -1];
        end
        if surfacenum == 18
            surface.bary = [0.2371, -0.4349, 0.2007]; % Converted from cm to m
            surface.size = 0.913944; % Converted from cm² to m²
            surface.unit = [0.5, -0.866, 0];
        end
        if surfacenum == 19
            surface.bary = [0.5362, -0.9530, -0.5808]; % Converted from cm to m
            surface.size = 0.690859; % Converted from cm² to m²
            surface.unit = [0, 0, 1];
        end
        if surfacenum == 20
            surface.bary = [0.5362, -0.9530, -0.6008]; % Converted from cm to m
            surface.size = 0.690859; % Converted from cm² to m²
            surface.unit = [0, 0, -1];
        end
        % 
        bary = R_princ*(surface.bary'); % Barycenter body to princ
        A = (surface.size); % Area in m^2
        N = R_princ*(surface.unit'); % Normal vector in princ
        % 
        % cos_theta_StoN = dot(N,V_p_unit); % Angle between N and V vectors
        theta_StoN = acos(dot(N, V_p_unit));

        % if cos_theta_StoN > 0 % Facing velocity or not 
        %     e = 1;
        % else
        %     e = 0;
        % end

        if theta_StoN >= 0 && theta_StoN <= pi/2
            e = 1; % Surfaces can see each other
        else
            e = 0; % Surfaces are obstructed
        end

        F = -(1/2)*C_d*A*rho*(norm(V_p)^2)*dot(V_p_unit,N)*V_p_unit; % Force
        M_aero = M_aero + cross(bary,F); % Summation 
    end
end

== matlab function mainEthan/Actuator and Control/Magnetorquer ==
  data: A input; I_w input; omega_w input; inertia_p input; omega input; B input; M_c output; m output; max_dipole input; noise input
%% return omega_dot (zero torque)
function [M_c, m]   = magnetorquer(A, I_w, omega_w, inertia_p, omega, B, max_dipole, noise)
    k = 0.003;
    
    H_D = A*(I_w*omega_w) + inertia_p * omega;
   
    m =  k/(norm(B)^2) * cross(H_D, B);
    m = max(min(m, max_dipole), -max_dipole) + noise';
    M_c = cross(m, B);
end

== matlab function mainEthan/Attitude Estimation/Deterministic Attitude Determination ==
  data: M input; V input; DCM_estimated output
%% return sensor measurements
function DCM_estimated = deterministic_attitude_determination(M, V)

    M_fict = M;
    V_fict = V;
    %generate fictitious measurement
    for i = 1:2:length(M(1, :))
        M_fict(:, i) = (M(:, i) + M(:, i+1))./2;
        V_fict(:, i) = (V(:, i) + V(:, i+1))./2;
        M_fict(:, i+1) = (M(:, i) - M(:, i+1))./2;
        V_fict(:, i+1) = (V(:, i) - V(:, i+1))./2;
    end


    DCM_estimated = M_fict * pinv(V_fict); %using fictitous measurements
    %DCM_estimated = M * pinv(V); %no fictitious measurements
        
end

== matlab function mainEthan/Orbit Propagation Sun 3.0/Approx ECI ==
  data: time_seconds input; state_sun_ECI output
function state_sun_ECI = our_approxECISunPosition(time_seconds)
% Given Gregorian year(s), day(s), and time(s), calculate Earth-centered
% inertial (ECI) coordinates (in meters) of the vector(s) pointing from
% Earth's center to the center of the Sun.
% Encapsulated by Seth B. Wagenman, from stargazing.net/kepler/sun.html as
% corrected by https://astronomy.stackexchange.com/a/37199/34646 along with
% other minor corrections based on recent revisions to the ecliptic plane.

% Convert seconds since epoch to MATLAB serial date number
time_seconds = squeeze(time_seconds);
MJD = 53029 + time_seconds/86400;
JD = MJD + 2400000.5;

% Convert MJD to datetime
% date_time = datetime(MJD, 'ConvertFrom', 'MJD');
% date_vector = datevec(date_time);


% Extract year, month, day, hour, minute, and second from datetime
% year_val = year(date_time);
% month_val = month(date_time);
% day_val = day(date_time);
% hour_val = hour(date_time);
% minute_val = minute(date_time);
% second_val = second(date_time);

% Create datetime vector
% dateTimeVector = [year_val, month_val, day_val, hour_val, minute_val, second_val];

% Set time(s) relative to the J2000.0 epoch
fractionalDay = JD - 2451545.0;

% Mean longitude of the Sun
meanLongitudeSunDegrees = 280.4606184 + ...
	((36000.77005361 / 36525) * fractionalDay); %(degrees)

% Mean anomaly of the Sun
meanAnomalySunDegrees = 357.5277233 + ...
	((35999.05034 / 36525) * fractionalDay); %(degrees)
meanAnomalySunRadians = meanAnomalySunDegrees * pi / 180;

% Ecliptic longitude of the Sun
eclipticLongitudeSunDegrees = meanLongitudeSunDegrees + ...
	(1.914666471 * sin(meanAnomalySunRadians)) + ...
	(0.918994643 * sin(2 * meanAnomalySunRadians)); %(degrees)
eclipticLongitudeSunRadians = eclipticLongitudeSunDegrees * pi / 180;

% Obliquity of the ecliptic plane formula mostly derived from:
% https://en.wikipedia.org/wiki/Ecliptic#Obliquity_of_the_ecliptic
epsilonDegrees = ... % Formula deals with time denominated in centuries
	23.43929 - ((46.8093 / 3600) * fractionalDay / 36525);  %(degrees)
epsilonRadians = epsilonDegrees * pi / 180;

% **** Calculations for unit vectors direction to the Sun are in ECI ****
% Now calculate the Earth to Sun unit vector(s) USING RADIANS, NOT DEGREES
unitEarthSunVectorTransposed = [cos(eclipticLongitudeSunRadians).';
    (cos(epsilonRadians) .* sin(eclipticLongitudeSunRadians)).';
    (sin(epsilonRadians) .* sin(eclipticLongitudeSunRadians)).'];
unitEarthSunVector = unitEarthSunVectorTransposed.';

% Scale up from unit vector(s); distances vary--Earth's orbit is elliptical
distEarthToSunInAstronomicalUnits = ...
	1.000140612 - ...
	(0.016708617 * cos(meanAnomalySunRadians)) - ...
	(0.000139589 * cos(2 * meanAnomalySunRadians)); % in Astronomical Units
distEarthToSunInMeters = ... % (new international definition for an A. U.)
	149597870700 * distEarthToSunInAstronomicalUnits;

% Multiply unit vector(s) by distance to Sun for scaling to full magnitude
state_sun_ECI = ... % Use meters for generic code compatibility
	(distEarthToSunInMeters .* unitEarthSunVector)/1000; 

end % End of function

== matlab function mainEthan/Attitude Estimation/MATLAB Function ==
  data: M input; quat_estimated output; V input
%% return estimated quaternions M = sun, magnet, star1, star2
function quat_estimated = Q_method(M, V)
    w_sun = 0.1;
    w_mag = 0.05;
    w_star =0.85;
    W = M;
    W(:,3:end) = sqrt(w_star).*M(:,3:end);
    W(:, 2) = sqrt(w_mag) .*M(:, 2);
    W(:, 1) = sqrt(w_sun) .*M(:, 1);

    U = V;
    U(:,3:end) = sqrt(w_star).*V(:,3:end);
    U(:, 2) = sqrt(w_mag) .*V(:, 2);
    U(:, 1) = sqrt(w_sun) .*V(:, 1);
 

    B = W*U';
    S = B + B';
    Z = [B(2,3) - B(3,2); B(3,1) - B(1,3); B(1,2)-B(2,1)];

    sigma = trace(B);

    K = [S - sigma*eye(3), Z; Z', sigma];
    [eigvec, eigval] = eig(K);
    eigenvalues = diag(eigval);

    [max_eigenvalue, max_index] = max(eigenvalues);

    max_eigvec = eigvec(:, max_index);

    quat_estimated = [real(max_eigvec(1)); real(max_eigvec(2)); real(max_eigvec(3)); real(max_eigvec(4))];
    quat_estimated = quat_estimated./norm(quat_estimated);
end
